simulink model "dp_EKF_ausschwing"  (R2015b)
settings: Solver=FixedStepAuto  StartTime=0.0  StopTime=5  FixedStep=T_s  RelTol=1e-3
values from neighbouring files (symbols this model uses):
  d_p1 = 0.001    [dp_EKF_anregung_script.m]    (also in dp_EKF_ausschwing_script.m; dp_UKF_anregung_script.m)
  d_p2 = 0.001    [dp_EKF_anregung_script.m]    (also in dp_EKF_ausschwing_script.m; dp_UKF_anregung_script.m)
  g = 9.81    [dp_EKF_anregung_script.m]    (also in dp_EKF_ausschwing_script.m; dp_UKF_anregung_script.m)
  i_min = i    [dp_EKF_anregung_script.m]    (also in dp_EKF_ausschwing_script.m)
  ii_min = ii    [dp_EKF_anregung_script.m]    (also in dp_EKF_ausschwing_script.m)
  l_1 = 0.194    [dp_EKF_anregung_script.m]    (also in dp_EKF_ausschwing_script.m; dp_UKF_anregung_script.m)
  l_2 = 0.1855    [dp_EKF_anregung_script.m]    (also in dp_EKF_ausschwing_script.m; dp_UKF_anregung_script.m)
  m_1 = 0.0313    [dp_EKF_anregung_script.m]    (also in dp_EKF_ausschwing_script.m; dp_UKF_anregung_script.m)
  m_2 = 0.0313    [dp_EKF_anregung_script.m]    (also in dp_EKF_ausschwing_script.m; dp_UKF_anregung_script.m)
  m_3 = 0.0308    [dp_EKF_anregung_script.m]    (also in dp_EKF_ausschwing_script.m; dp_UKF_anregung_script.m)
  Pk_0 = eye(4)    [dp_EKF_anregung_script.m]    (also in dp_EKF_ausschwing_script.m; dp_UKF_anregung_script.m = 10*eye(4))
  Qk = zeros(4,4,steps,steps,steps,steps)    [dp_EKF_anregung_script.m]    (also in dp_EKF_ausschwing_script.m = zeros(4,4,steps,steps); dp_UKF_anregung_script.m = zeros(4,4,4,4))
  Qk_min = diag([0.0001 1 0.1 10])    [dp_EKF_anregung_script.m]    (also in dp_EKF_ausschwing_script.m = Qk(:,:,i,ii))
  Rk = 1    [dp_EKF_anregung_script.m]    (also in dp_EKF_ausschwing_script.m; dp_UKF_anregung_script.m)
  T_s = 0.001    [dp_EKF_anregung_script.m]    (also in dp_EKF_ausschwing_script.m; dp_UKF_anregung_script.m)
  x0_ekf = x0    [dp_EKF_anregung_script.m]    (also in dp_EKF_ausschwing_script.m = [-30*0.0175; 5; 30*0.0175; -4])
libraries: simulink x2
settings Model: Creator=serov  LastModifiedBy=serov
settings DataIOCC: LimitDataPoints=off

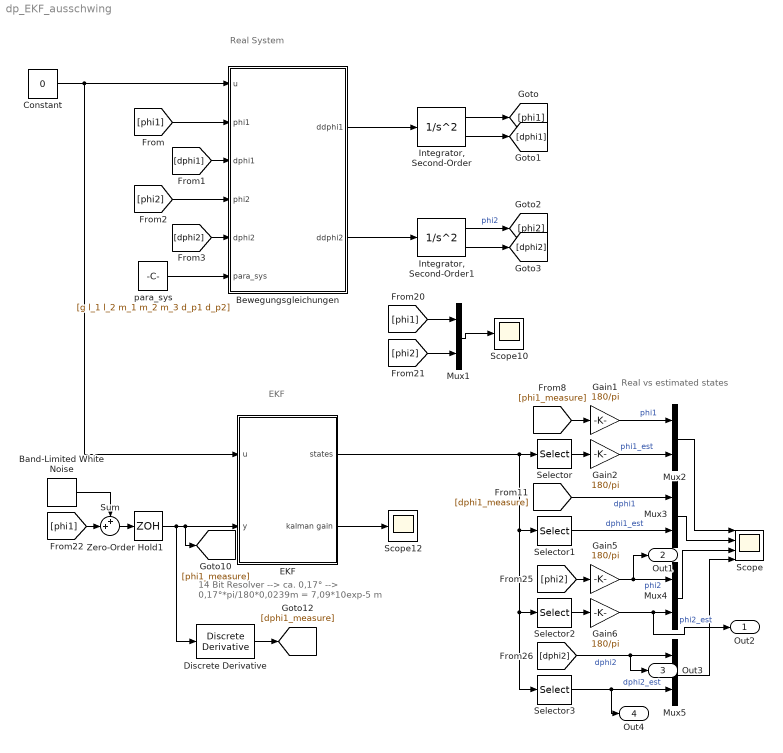
== system dp_EKF_ausschwing ==
  note: Real vs estimated states
  note: Real System
  note: EKF
  note: 14 Bit Resolver --> ca. 0,17°
      | --> 0,17°*pi/180*0,0239m = 7,09*10exp-5 m
  Band-Limited White Noise : simulink/Sources/Band-Limited White Noise  Cov=noise_power  Ts=T_s  seed=[23341]
  Bewegungsgleichungen : MATLAB Function  TreatAsAtomicUnit=on
  Constant : Constant  Value=0
  Discrete Derivative : simulink/Discrete/Discrete Derivative  gainval=1.0  ICPrevScaledInput=0.0  InputProcessing=Inherited  OutMin=[]  OutMax=[]  OutDataType=fixdt(1, 16)  OutScaling=2^-10  DoSatur=off
  EKF : Subsystem
  Gain{1..2,5..6} (4 alike) : Gain  Gain=180/pi
  "Integrator, Second-Order" : SecondOrderIntegrator  ICX=phi1_0  ICDXDT=dphi1_0
  "Integrator, Second-Order1" : SecondOrderIntegrator  ICX=phi2_0  ICDXDT=dphi2_0
  Mux{1..5} (5 alike) : Mux  Inputs=2
  Scope : Scope  NumInputPorts=4
  Scope10 : Scope
  Scope12 : Scope
  Selector : Selector  InputPortWidth=4  IndexOptions=Index vector (dialog)  Indices=[1]  OutputSizes=1
  Selector1 : Selector  InputPortWidth=4  IndexOptions=Index vector (dialog)  Indices=[2]  OutputSizes=1
  Selector2 : Selector  InputPortWidth=4  IndexOptions=Index vector (dialog)  Indices=[3]  OutputSizes=1
  Selector3 : Selector  InputPortWidth=4  IndexOptions=Index vector (dialog)  Indices=[4]  OutputSizes=1
  Sum : Sum  Inputs=++|
  Zero-Order Hold1 : ZeroOrderHold  SampleTime=T_s
  para_sys : Constant  Value=[g l_1 l_2 m_1 m_2 m_3 d_p1 d_p2]
  Out2 : Outport
  Out1 : Outport  Port=2
  Out3 : Outport  Port=3
  Out4 : Outport  Port=4
  wires:
  Bewegungsgleichungen/1(ddphi1) -> "Integrator, Second-Order"/1
  Bewegungsgleichungen/2(ddphi2) -> "Integrator, Second-Order1"/1
  "Integrator, Second-Order"/2 -> [dphi1]
  "Integrator, Second-Order1"/2 -> [dphi2]
  [phi1] -> Bewegungsgleichungen/2(phi1)
  [dphi1] -> Bewegungsgleichungen/3(dphi1)
  [phi2] -> Bewegungsgleichungen/4(phi2)
  [dphi2] -> Bewegungsgleichungen/5(dphi2)
  para_sys/1 -> Bewegungsgleichungen/6(para_sys)
  Mux1/1 -> Scope10/1
  [phi2] -> Mux1/2
  EKF/2(kalman gain) -> Scope12/1
  Zero-Order Hold1/1 -> Discrete Derivative/1, [phi1_measure], EKF/2(y)
  Gain1/1 -> Mux2/1  "phi1"
  Gain2/1 -> Mux2/2  "phi1_est"
  Selector/1 -> Gain2/1
  [dphi1_measure] -> Mux3/1  "dphi1"
  Selector1/1 -> Mux3/2  "dphi1_est"
  [phi2] -> Gain5/1
  Gain5/1 -> Out1/1, Mux4/1  "phi2"
  Gain6/1 -> Out2/1, Mux4/2  "phi2_est"
  Selector2/1 -> Gain6/1
  [dphi2] -> Out3/1, Mux5/1  "dphi2"
  Selector3/1 -> Out4/1, Mux5/2  "dphi2_est"
  EKF/1(states) -> Selector3/1, Selector2/1, Selector1/1, Selector/1
  Mux2/1 -> Scope/1
  Mux3/1 -> Scope/2
  Mux5/1 -> Scope/4
  [phi1] -> Sum/2
  Band-Limited White Noise/1 -> Sum/1
  Sum/1 -> Zero-Order Hold1/1
  "Integrator, Second-Order"/1 -> [phi1]
  Discrete Derivative/1 -> [dphi1_measure]
  Mux4/1 -> Scope/3
  Constant/1 -> EKF/1(u), Bewegungsgleichungen/1(u)
  [phi1_measure] -> Gain1/1
  [phi1] -> Mux1/1
  "Integrator, Second-Order1"/1 -> [phi2]  "phi2"

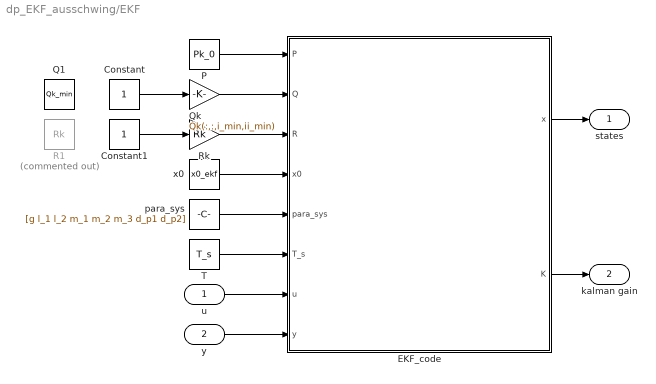
== system dp_EKF_ausschwing/EKF ==
  u : Inport
  y : Inport  Port=2
  Constant : Constant
  Constant1 : Constant
  EKF_code : MATLAB Function  TreatAsAtomicUnit=on
  P : Constant  Value=Pk_0
  Q1 : Constant  Value=Qk_min
  Qk : Gain  Gain=Qk(:,:,i_min,ii_min)
  R1 : Constant  Commented=on  Value=Rk
  Rk : Gain  Gain=Rk
  T : Constant  Value=T_s
  para_sys : Constant  Value=[g l_1 l_2 m_1 m_2 m_3 d_p1 d_p2]
  x0 : Constant  Value=x0_ekf
  states : Outport
  kalman gain : Outport  Port=2
  wires:
  P/1 -> EKF_code/1(P)
  Rk/1 -> EKF_code/3(R)
  x0/1 -> EKF_code/4(x0)
  para_sys/1 -> EKF_code/5(para_sys)
  T/1 -> EKF_code/6(T_s)
  u/1 -> EKF_code/7(u)
  y/1 -> EKF_code/8(y)
  EKF_code/1(x) -> states/1
  EKF_code/2(K) -> kalman gain/1
  Constant/1 -> Qk/1
  Constant1/1 -> Rk/1
  Qk/1 -> EKF_code/2(Q)

== matlab function dp_EKF_ausschwing/EKF/EKF_code ==
  data: P input; Q input; R input; x0 input; para_sys input; T_s input; u input; y input; x output; K output
function [x, K]  = extended_kalman_filter(P, Q, R, x0, para_sys, T_s, u, y)
% Extended Kalman Filter (EKF) fuer nichtlineare Systeme
% Das Extended Kalman Filter praediziert den Zustand eines nichtlinearen
% Systems durch Linearisierung im Arbeistpunkt.
% R ist die Kovarianzmatrix fuer das Messrauschen.
% Q ist die Kovarianzmatrix fuer das Prozessrauschen.
% Das Verhaeltnis von Q und R gibt die Dynamik des Filters vor.

persistent x_p P_p
% Parameter

g = para_sys(1);
l_1 = para_sys(2);
l_2 = para_sys(3);
m_1 = para_sys(4);
m_2 = para_sys(5);
m_3 = para_sys(6);
d_p1 = para_sys(7);
d_p2 = para_sys(8);

if isempty(x_p)
   x_p = x0;
%    x_p = [0*0.0175; 0; 0.0175;0];
   P_p = P;
   x = x_p;
   K = zeros(4,1);
else
%% Discrete Kalman filter time update equations

 x_1 = x_p(1);
 x_2 = x_p(2);
 x_3 = x_p(3);
 x_4 = x_p(4);

x = [x_1 + T_s*x_2;x_2 + (T_s*(12*d_p2*l_2*x_4 - 12*d_p1*l_2*x_2 - 12*d_p2*l_2*x_2 - cos(x_1 - x_3)*(18*d_p2*l_1*x_2 - 18*d_p2*l_1*x_4 + 9*l_1*l_2*m_2*u*cos(x_3) + 9*g*l_1*l_2*m_2*sin(x_3) + 9*l_1^2*l_2*m_2*x_2^2*sin(x_1 - x_3)) + 6*l_1*l_2*m_1*u*cos(x_1) + 12*l_1*l_2*m_2*u*cos(x_1) + 12*l_1*l_2*m_3*u*cos(x_1) + 6*g*l_1*l_2*m_1*sin(x_1) + 12*g*l_1*l_2*m_2*sin(x_1) + 12*g*l_1*l_2*m_3*sin(x_1) - 6*l_1*l_2^2*m_2*x_4^2*sin(x_1 - x_3)))/(l_1^2*l_2*(4*m_1 + 12*m_2 + 12*m_3 - 9*m_2*cos(x_1 - x_3)^2));x_3 + T_s*x_4;x_4 + (T_s*(sin(x_1 - x_3)*(36*l_1^2*l_2*m_2^2*x_2^2 + 12*l_1^2*l_2*m_1*m_2*x_2^2 + 36*l_1^2*l_2*m_2*m_3*x_2^2) + 24*d_p2*l_1*m_1*x_2 + 72*d_p2*l_1*m_2*x_2 - 24*d_p2*l_1*m_1*x_4 + 72*d_p2*l_1*m_3*x_2 - 72*d_p2*l_1*m_2*x_4 - 72*d_p2*l_1*m_3*x_4 + 36*d_p1*l_2*m_2*x_2*cos(x_1 - x_3) + 36*d_p2*l_2*m_2*x_2*cos(x_1 - x_3) - 36*d_p2*l_2*m_2*x_4*cos(x_1 - x_3) + 18*l_1*l_2*m_2^2*u*cos(x_3) + 18*g*l_1*l_2*m_2^2*sin(x_3) + 9*l_1*l_2^2*m_2^2*x_4^2*sin(2*x_1 - 2*x_3) - 18*l_1*l_2*m_2^2*u*cos(2*x_1 - x_3) - 18*g*l_1*l_2*m_2^2*sin(2*x_1 - x_3) + 3*l_1*l_2*m_1*m_2*u*cos(x_3) + 18*l_1*l_2*m_2*m_3*u*cos(x_3) + 3*g*l_1*l_2*m_1*m_2*sin(x_3) + 18*g*l_1*l_2*m_2*m_3*sin(x_3) - 9*l_1*l_2*m_1*m_2*u*cos(2*x_1 - x_3) - 18*l_1*l_2*m_2*m_3*u*cos(2*x_1 - x_3) - 9*g*l_1*l_2*m_1*m_2*sin(2*x_1 - x_3) - 18*g*l_1*l_2*m_2*m_3*sin(2*x_1 - x_3)))/(l_1*l_2^2*m_2*(8*m_1 + 15*m_2 + 24*m_3 - 9*m_2*cos(2*x_1 - 2*x_3)))];
       
        % Jacobian Matrix
A = [1, T_s, 0, 0;- (T_s*(6*l_1*l_2*m_1*u*sin(x_1) - sin(x_1 - x_3)*(18*d_p2*l_1*x_2 - 18*d_p2*l_1*x_4 + 9*l_1*l_2*m_2*u*cos(x_3) + 9*g*l_1*l_2*m_2*sin(x_3) + 9*l_1^2*l_2*m_2*x_2^2*sin(x_1 - x_3)) + 12*l_1*l_2*m_2*u*sin(x_1) + 12*l_1*l_2*m_3*u*sin(x_1) + 9*l_1^2*l_2*m_2*x_2^2*cos(x_1 - x_3)^2 - 6*g*l_1*l_2*m_1*cos(x_1) - 12*g*l_1*l_2*m_2*cos(x_1) - 12*g*l_1*l_2*m_3*cos(x_1) + 6*l_1*l_2^2*m_2*x_4^2*cos(x_1 - x_3)))/(l_1^2*l_2*(4*m_1 + 12*m_2 + 12*m_3 - 9*m_2*cos(x_1 - x_3)^2)) - (18*T_s*m_2*cos(x_1 - x_3)*sin(x_1 - x_3)*(12*d_p2*l_2*x_4 - 12*d_p1*l_2*x_2 - 12*d_p2*l_2*x_2 - cos(x_1 - x_3)*(18*d_p2*l_1*x_2 - 18*d_p2*l_1*x_4 + 9*l_1*l_2*m_2*u*cos(x_3) + 9*g*l_1*l_2*m_2*sin(x_3) + 9*l_1^2*l_2*m_2*x_2^2*sin(x_1 - x_3)) + 6*l_1*l_2*m_1*u*cos(x_1) + 12*l_1*l_2*m_2*u*cos(x_1) + 12*l_1*l_2*m_3*u*cos(x_1) + 6*g*l_1*l_2*m_1*sin(x_1) + 12*g*l_1*l_2*m_2*sin(x_1) + 12*g*l_1*l_2*m_3*sin(x_1) - 6*l_1*l_2^2*m_2*x_4^2*sin(x_1 - x_3)))/(l_1^2*l_2*(4*m_1 + 12*m_2 + 12*m_3 - 9*m_2*cos(x_1 - x_3)^2)^2), 1 - (T_s*(12*d_p1*l_2 + 12*d_p2*l_2 + cos(x_1 - x_3)*(18*d_p2*l_1 + 18*l_1^2*l_2*m_2*x_2*sin(x_1 - x_3))))/(l_1^2*l_2*(4*m_1 + 12*m_2 + 12*m_3 - 9*m_2*cos(x_1 - x_3)^2)), (T_s*(cos(x_1 - x_3)*(9*l_1*l_2*m_2*u*sin(x_3) - 9*g*l_1*l_2*m_2*cos(x_3) + 9*l_1^2*l_2*m_2*x_2^2*cos(x_1 - x_3)) - sin(x_1 - x_3)*(18*d_p2*l_1*x_2 - 18*d_p2*l_1*x_4 + 9*l_1*l_2*m_2*u*cos(x_3) + 9*g*l_1*l_2*m_2*sin(x_3) + 9*l_1^2*l_2*m_2*x_2^2*sin(x_1 - x_3)) + 6*l_1*l_2^2*m_2*x_4^2*cos(x_1 - x_3)))/(l_1^2*l_2*(4*m_1 + 12*m_2 + 12*m_3 - 9*m_2*cos(x_1 - x_3)^2)) + (18*T_s*m_2*cos(x_1 - x_3)*sin(x_1 - x_3)*(12*d_p2*l_2*x_4 - 12*d_p1*l_2*x_2 - 12*d_p2*l_2*x_2 - cos(x_1 - x_3)*(18*d_p2*l_1*x_2 - 18*d_p2*l_1*x_4 + 9*l_1*l_2*m_2*u*cos(x_3) + 9*g*l_1*l_2*m_2*sin(x_3) + 9*l_1^2*l_2*m_2*x_2^2*sin(x_1 - x_3)) + 6*l_1*l_2*m_1*u*cos(x_1) + 12*l_1*l_2*m_2*u*cos(x_1) + 12*l_1*l_2*m_3*u*cos(x_1) + 6*g*l_1*l_2*m_1*sin(x_1) + 12*g*l_1*l_2*m_2*sin(x_1) + 12*g*l_1*l_2*m_3*sin(x_1) - 6*l_1*l_2^2*m_2*x_4^2*sin(x_1 - x_3)))/(l_1^2*l_2*(4*m_1 + 12*m_2 + 12*m_3 - 9*m_2*cos(x_1 - x_3)^2)^2), (T_s*(12*d_p2*l_2 + 18*d_p2*l_1*cos(x_1 - x_3) - 12*l_1*l_2^2*m_2*x_4*sin(x_1 - x_3)))/(l_1^2*l_2*(4*m_1 + 12*m_2 + 12*m_3 - 9*m_2*cos(x_1 - x_3)^2));0, 0, 1, T_s;(T_s*(cos(x_1 - x_3)*(36*l_1^2*l_2*m_2^2*x_2^2 + 12*l_1^2*l_2*m_1*m_2*x_2^2 + 36*l_1^2*l_2*m_2*m_3*x_2^2) - 36*d_p1*l_2*m_2*x_2*sin(x_1 - x_3) - 36*d_p2*l_2*m_2*x_2*sin(x_1 - x_3) + 36*d_p2*l_2*m_2*x_4*sin(x_1 - x_3) + 18*l_1*l_2^2*m_2^2*x_4^2*cos(2*x_1 - 2*x_3) - 36*g*l_1*l_2*m_2^2*cos(2*x_1 - x_3) + 36*l_1*l_2*m_2^2*u*sin(2*x_1 - x_3) + 18*l_1*l_2*m_1*m_2*u*sin(2*x_1 - x_3) + 36*l_1*l_2*m_2*m_3*u*sin(2*x_1 - x_3) - 18*g*l_1*l_2*m_1*m_2*cos(2*x_1 - x_3) - 36*g*l_1*l_2*m_2*m_3*cos(2*x_1 - x_3)))/(l_1*l_2^2*m_2*(8*m_1 + 15*m_2 + 24*m_3 - 9*m_2*cos(2*x_1 - 2*x_3))) - (18*T_s*sin(2*x_1 - 2*x_3)*(sin(x_1 - x_3)*(36*l_1^2*l_2*m_2^2*x_2^2 + 12*l_1^2*l_2*m_1*m_2*x_2^2 + 36*l_1^2*l_2*m_2*m_3*x_2^2) + 24*d_p2*l_1*m_1*x_2 + 72*d_p2*l_1*m_2*x_2 - 24*d_p2*l_1*m_1*x_4 + 72*d_p2*l_1*m_3*x_2 - 72*d_p2*l_1*m_2*x_4 - 72*d_p2*l_1*m_3*x_4 + 36*d_p1*l_2*m_2*x_2*cos(x_1 - x_3) + 36*d_p2*l_2*m_2*x_2*cos(x_1 - x_3) - 36*d_p2*l_2*m_2*x_4*cos(x_1 - x_3) + 18*l_1*l_2*m_2^2*u*cos(x_3) + 18*g*l_1*l_2*m_2^2*sin(x_3) + 9*l_1*l_2^2*m_2^2*x_4^2*sin(2*x_1 - 2*x_3) - 18*l_1*l_2*m_2^2*u*cos(2*x_1 - x_3) - 18*g*l_1*l_2*m_2^2*sin(2*x_1 - x_3) + 3*l_1*l_2*m_1*m_2*u*cos(x_3) + 18*l_1*l_2*m_2*m_3*u*cos(x_3) + 3*g*l_1*l_2*m_1*m_2*sin(x_3) + 18*g*l_1*l_2*m_2*m_3*sin(x_3) - 9*l_1*l_2*m_1*m_2*u*cos(2*x_1 - x_3) - 18*l_1*l_2*m_2*m_3*u*cos(2*x_1 - x_3) - 9*g*l_1*l_2*m_1*m_2*sin(2*x_1 - x_3) - 18*g*l_1*l_2*m_2*m_3*sin(2*x_1 - x_3)))/(l_1*l_2^2*(8*m_1 + 15*m_2 + 24*m_3 - 9*m_2*cos(2*x_1 - 2*x_3))^2), (T_s*(sin(x_1 - x_3)*(72*l_1^2*l_2*m_2^2*x_2 + 24*l_1^2*l_2*m_1*m_2*x_2 + 72*l_1^2*l_2*m_2*m_3*x_2) + 24*d_p2*l_1*m_1 + 72*d_p2*l_1*m_2 + 72*d_p2*l_1*m_3 + 36*d_p1*l_2*m_2*cos(x_1 - x_3) + 36*d_p2*l_2*m_2*cos(x_1 - x_3)))/(l_1*l_2^2*m_2*(8*m_1 + 15*m_2 + 24*m_3 - 9*m_2*cos(2*x_1 - 2*x_3))), (18*T_s*sin(2*x_1 - 2*x_3)*(sin(x_1 - x_3)*(36*l_1^2*l_2*m_2^2*x_2^2 + 12*l_1^2*l_2*m_1*m_2*x_2^2 + 36*l_1^2*l_2*m_2*m_3*x_2^2) + 24*d_p2*l_1*m_1*x_2 + 72*d_p2*l_1*m_2*x_2 - 24*d_p2*l_1*m_1*x_4 + 72*d_p2*l_1*m_3*x_2 - 72*d_p2*l_1*m_2*x_4 - 72*d_p2*l_1*m_3*x_4 + 36*d_p1*l_2*m_2*x_2*cos(x_1 - x_3) + 36*d_p2*l_2*m_2*x_2*cos(x_1 - x_3) - 36*d_p2*l_2*m_2*x_4*cos(x_1 - x_3) + 18*l_1*l_2*m_2^2*u*cos(x_3) + 18*g*l_1*l_2*m_2^2*sin(x_3) + 9*l_1*l_2^2*m_2^2*x_4^2*sin(2*x_1 - 2*x_3) - 18*l_1*l_2*m_2^2*u*cos(2*x_1 - x_3) - 18*g*l_1*l_2*m_2^2*sin(2*x_1 - x_3) + 3*l_1*l_2*m_1*m_2*u*cos(x_3) + 18*l_1*l_2*m_2*m_3*u*cos(x_3) + 3*g*l_1*l_2*m_1*m_2*sin(x_3) + 18*g*l_1*l_2*m_2*m_3*sin(x_3) - 9*l_1*l_2*m_1*m_2*u*cos(2*x_1 - x_3) - 18*l_1*l_2*m_2*m_3*u*cos(2*x_1 - x_3) - 9*g*l_1*l_2*m_1*m_2*sin(2*x_1 - x_3) - 18*g*l_1*l_2*m_2*m_3*sin(2*x_1 - x_3)))/(l_1*l_2^2*(8*m_1 + 15*m_2 + 24*m_3 - 9*m_2*cos(2*x_1 - 2*x_3))^2) - (T_s*(cos(x_1 - x_3)*(36*l_1^2*l_2*m_2^2*x_2^2 + 12*l_1^2*l_2*m_1*m_2*x_2^2 + 36*l_1^2*l_2*m_2*m_3*x_2^2) - 36*d_p1*l_2*m_2*x_2*sin(x_1 - x_3) - 36*d_p2*l_2*m_2*x_2*sin(x_1 - x_3) + 36*d_p2*l_2*m_2*x_4*sin(x_1 - x_3) - 18*g*l_1*l_2*m_2^2*cos(x_3) + 18*l_1*l_2*m_2^2*u*sin(x_3) + 18*l_1*l_2^2*m_2^2*x_4^2*cos(2*x_1 - 2*x_3) - 18*g*l_1*l_2*m_2^2*cos(2*x_1 - x_3) + 18*l_1*l_2*m_2^2*u*sin(2*x_1 - x_3) + 9*l_1*l_2*m_1*m_2*u*sin(2*x_1 - x_3) + 18*l_1*l_2*m_2*m_3*u*sin(2*x_1 - x_3) - 3*g*l_1*l_2*m_1*m_2*cos(x_3) - 18*g*l_1*l_2*m_2*m_3*cos(x_3) + 3*l_1*l_2*m_1*m_2*u*sin(x_3) + 18*l_1*l_2*m_2*m_3*u*sin(x_3) - 9*g*l_1*l_2*m_1*m_2*cos(2*x_1 - x_3) - 18*g*l_1*l_2*m_2*m_3*cos(2*x_1 - x_3)))/(l_1*l_2^2*m_2*(8*m_1 + 15*m_2 + 24*m_3 - 9*m_2*cos(2*x_1 - 2*x_3))), 1 - (T_s*(24*d_p2*l_1*m_1 + 72*d_p2*l_1*m_2 + 72*d_p2*l_1*m_3 + 36*d_p2*l_2*m_2*cos(x_1 - x_3) - 18*l_1*l_2^2*m_2^2*x_4*sin(2*x_1 - 2*x_3)))/(l_1*l_2^2*m_2*(8*m_1 + 15*m_2 + 24*m_3 - 9*m_2*cos(2*x_1 - 2*x_3)))];
C = [1 0 0 0];

%% Discrete Kalman filter measurement update equations
P   = A * P_p * A' + Q;
K   = P * C'/( C * P * C' + R);
x   = x + (K * (y - C * x));
P_p  = (eye(size(A)) - K * C) * P;

x_p  = x;
end

== matlab function dp_EKF_ausschwing/Bewegungsgleichungen ==
  data: u input; phi1 input; dphi1 input; phi2 input; dphi2 input; para_sys input; ddphi1 output; ddphi2 output
function [ddphi1, ddphi2] = pendel_1_2(u, phi1, dphi1, phi2, dphi2, para_sys)
%#codegen

g = para_sys(1);
l_1 = para_sys(2);
l_2 = para_sys(3);
m_1 = para_sys(4);
m_2 = para_sys(5);
m_3 = para_sys(6);
d_p1 = para_sys(7);
d_p2 = para_sys(8);

ddphi1 = 1/(l_1^2*(9*cos(phi1-phi2)^2*m_2-4*m_1-12*m_2-12*m_3)*l_2)*(9*dphi1^2*cos(phi1-phi2)*sin(phi1-phi2)*l_1^2*l_2*m_2+6*m_2*l_1*l_2^2*sin(phi1-phi2)*dphi2^2+9*u*cos(phi1-phi2)*cos(phi2)*l_1*l_2*m_2+9*cos(phi1-phi2)*sin(phi2)*g*l_1*l_2*m_2-6*l_1*cos(phi1)*u*m_1*l_2-12*l_1*cos(phi1)*u*m_2*l_2-12*l_1*cos(phi1)*u*m_3*l_2-6*l_1*g*sin(phi1)*m_1*l_2-12*l_1*g*sin(phi1)*m_2*l_2-12*l_1*g*sin(phi1)*m_3*l_2+18*dphi1*cos(phi1-phi2)*d_p2*l_1-18*dphi2*cos(phi1-phi2)*d_p2*l_1+12*dphi1*d_p1*l_2+12*dphi1*d_p2*l_2-12*d_p2*dphi2*l_2);

ddphi2 = -1/(l_1*l_2^2*(9*cos(phi1-phi2)^2*m_2-4*m_1-12*m_2-12*m_3)*m_2)*(12*dphi1*d_p2*l_1*m_1+36*dphi1*d_p2*l_1*m_2+36*dphi1*d_p2*l_1*m_3-12*dphi2*d_p2*l_1*m_1-36*dphi2*d_p2*l_1*m_2-36*dphi2*d_p2*l_1*m_3-9*cos(phi1)*u*cos(phi1-phi2)*l_1*l_2*m_1*m_2-18*cos(phi1)*u*cos(phi1-phi2)*l_1*l_2*m_2*m_3-9*cos(phi1-phi2)*sin(phi1)*g*l_1*l_2*m_1*m_2-18*cos(phi1-phi2)*sin(phi1)*g*l_1*l_2*m_2*m_3+9*dphi2^2*cos(phi1-phi2)*sin(phi1-phi2)*l_1*l_2^2*m_2^2+ 6*dphi1^2*sin(phi1-phi2)*l_1^2*l_2*m_1*m_2+ 18*dphi1^2*sin(phi1-phi2)*l_1^2*l_2*m_2*m_3-18*cos(phi1)*u*cos(phi1-phi2)*l_1*l_2*m_2^2-18*cos(phi1-phi2)*sin(phi1)*g*l_1*l_2*m_2^2 +6*u*cos(phi2)*l_1*l_2*m_1*m_2+18*u*cos(phi2)*l_1*l_2*m_2*m_3+6*sin(phi2)*g*l_1*l_2*m_1*m_2+18*sin(phi2)*g*l_1*l_2*m_2*m_3 + 18*(dphi1)^2*sin(phi1-phi2)*l_1^2*l_2*m_2^2+18*u*cos(phi2)*l_1*l_2*m_2^2+18*sin(phi2)*g*l_1*l_2*m_2^2+18*dphi1*cos(phi1-phi2)*d_p1*l_2*m_2 + 18*dphi1*cos(phi1-phi2)*d_p2*l_2*m_2-18*dphi2*cos(phi1-phi2)*d_p2*l_2*m_2);
